simulink model "Quaternions_Method"  (R2021b)
settings: Solver=ode113  StartTime=0.0  StopTime=Time  RelTol=1e-13  AbsTol=1e-8
values from neighbouring files (symbols this model uses):
  a = 8.6251e+06    (= 8625100)    [Quaternions_method_parameters.m]    (also in car2kep.m = -(mu/(2*E)))
  A_MB = 0.5    [Quaternions_method_parameters.m]
  A_SP = 1    [Quaternions_method_parameters.m]
  c = 299792*10^3    (= 299792000)    [Quaternions_method_parameters.m]
  e = norm(e)    [Lab_7_task_1_4_parameters.m]    (also in Lab_7_task_5_parameters.m; Quaternions_method_parameters.m = 0.1195; car2kep.m = 1/mu * [((v_norm)^2 - (mu/r_norm)).*r - (dot(r, v).*v)])
  ii = 0.3815    [Quaternions_method_parameters.m]
  Ix = 0.04    [Quaternions_method_parameters.m]
  Iy = 0.06    [Quaternions_method_parameters.m]
  Iz = 0.08    [Quaternions_method_parameters.m]
  muP = astroConstants(13)*10^9    [Lab_7_task_1_4_parameters.m]    (also in Lab_7_task_5_parameters.m; Quaternions_method_parameters.m = 398527110340000)
  om_x = 1e-6    (= 1e-06)    [Quaternions_method_parameters.m]
  om_y = 1e-6    (= 1e-06)    [Quaternions_method_parameters.m]
  om_z = n    [Quaternions_method_parameters.m]
  omega_0 = [om_x, om_y, om_z]    [Quaternions_method_parameters.m]
  RS_MB = 0.5    [Quaternions_method_parameters.m]
  theta00 = 0    [Quaternions_method_parameters.m]
undefined symbols (not defined in the file or in its folder): I, Iinv, Rs_SP
libraries: vrlib x3, simulink_extras x1, robotcorelib x1
(part 2 of 2)

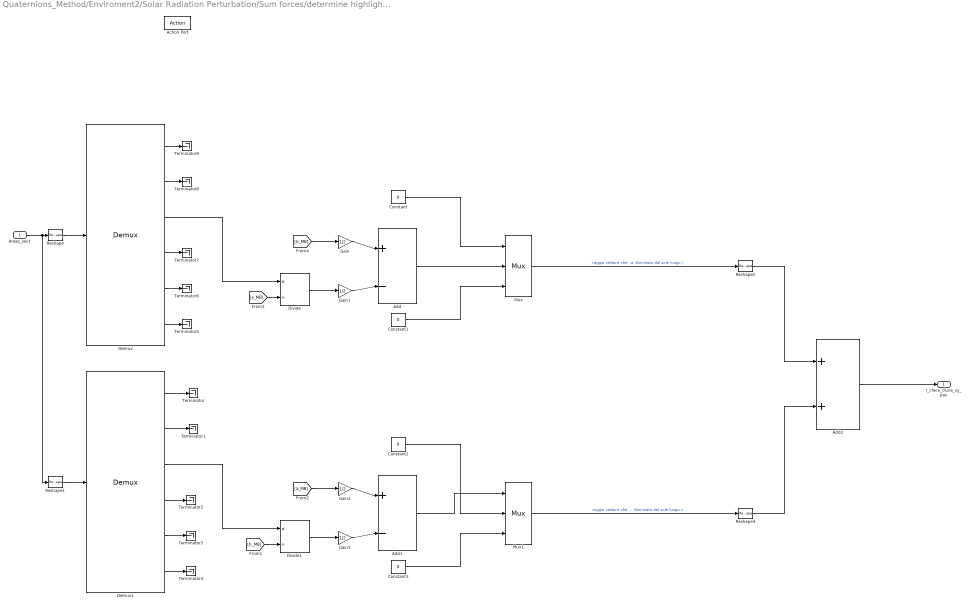
== system Quaternions_Method/Enviroment2/Solar Radiation Perturbation/Sum forces/determine highlighted area/creazione della matrice che ha per colonne i vettori distanza tra il CM del MB e i centri geom delle aree illuminate dal sole /If Action Subsystem ==
  Areas_vect : Inport
  Action Port : ActionPort  ActionPortLabel=if(u1>0 & u2>0)
  Add : Sum  Inputs=+|-
  Add1 : Sum  Inputs=+|-
  Add2 : Sum
  Constant{,1..3} (4 alike) : Constant  Value=0
  Demux : Demux  Outputs=6
  Demux1 : Demux  Outputs=6
  Divide : Product  Inputs=*/
  Divide1 : Product  Inputs=*/
  Gain{,1..3} (4 alike) : Gain  Gain=1/2
  Mux : Mux  Inputs=3
  Mux1 : Mux  Inputs=3
  Reshape{,1..3} (4 alike) : Reshape  OutputDimensionality=Column vector (2-D)
  Terminator{,1..9} (10 alike) : Terminator
  r_cface_cluce_xy_pos : Outport
  wires:
  Constant/1 -> Mux/1
  Add/1 -> Mux/2
  Divide/1 -> Gain1/1
  Mux/1 -> Reshape2/1  "raggio vettore che collega il centro geom della faccia con il centro geom della faccia illuminata dal sole lungo j"
  Gain1/1 -> Add/2
  Demux/3 -> Divide/1
  [b_MB] -> Gain/1
  Gain/1 -> Add/1
  [a_MB] -> Divide/2
  Areas_vect/1 -> Reshape1/1, Reshape/1
  Constant1/1 -> Mux/3
  Reshape/1 -> Demux/1
  Add1/1 -> Mux1/1
  [b_MB] -> Divide1/2
  Mux1/1 -> Reshape3/1  "raggio vettore che collega il centro geom della faccia con il centro geom della faccia illuminata dal sole lungo x"
  Constant2/1 -> Mux1/2
  Demux1/3 -> Divide1/1
  Constant3/1 -> Mux1/3
  Gain3/1 -> Add1/2
  Gain2/1 -> Add1/1
  Reshape1/1 -> Demux1/1
  Divide1/1 -> Gain3/1
  [a_MB] -> Gain2/1
  Reshape2/1 -> Add2/1
  Reshape3/1 -> Add2/2
  Add2/1 -> r_cface_cluce_xy_pos/1
  Demux1/1 -> Terminator/1
  Demux1/2 -> Terminator1/1
  Demux1/5 -> Terminator3/1
  Demux1/6 -> Terminator4/1
  Demux1/4 -> Terminator2/1
  Demux/6 -> Terminator5/1
  Demux/5 -> Terminator6/1
  Demux/4 -> Terminator7/1
  Demux/1 -> Terminator9/1
  Demux/2 -> Terminator8/1

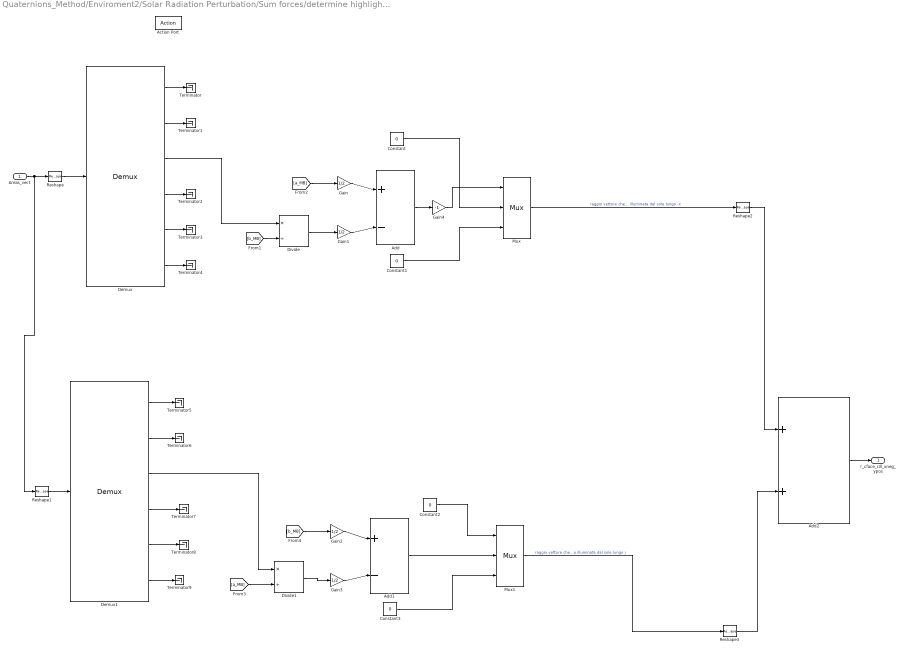
== system Quaternions_Method/Enviroment2/Solar Radiation Perturbation/Sum forces/determine highlighted area/creazione della matrice che ha per colonne i vettori distanza tra il CM del MB e i centri geom delle aree illuminate dal sole /If Action Subsystem1 ==
  Areas_vect : Inport
  Action Port : ActionPort  ActionPortLabel=if(u1<0 & u2>0)
  Add : Sum  Inputs=+|-
  Add1 : Sum  Inputs=+|-
  Add2 : Sum
  Constant{,1..3} (4 alike) : Constant  Value=0
  Demux : Demux  Outputs=6
  Demux1 : Demux  Outputs=6
  Divide : Product  Inputs=*/
  Divide1 : Product  Inputs=*/
  Gain{,1..3} (4 alike) : Gain  Gain=1/2
  Gain4 : Gain  Gain=-1
  Mux : Mux  Inputs=3
  Mux1 : Mux  Inputs=3
  Reshape{,1..3} (4 alike) : Reshape  OutputDimensionality=Column vector (2-D)
  Terminator{,1..9} (10 alike) : Terminator
  r_cface_cill_xneg_ypos : Outport
  wires:
  Reshape2/1 -> Add2/1
  Areas_vect/1 -> Reshape1/1, Reshape/1
  [b_MB] -> Divide/2
  Reshape/1 -> Demux/1
  [a_MB] -> Gain/1
  Gain/1 -> Add/1
  Gain1/1 -> Add/2
  Constant1/1 -> Mux/3
  Mux/1 -> Reshape2/1  "raggio vettore che collega il centro geom della faccia con il centro geom della faccia illuminata dal sole lungo -x"
  Demux/3 -> Divide/1
  Divide/1 -> Gain1/1
  Constant/1 -> Mux/2
  Reshape3/1 -> Add2/2
  Constant2/1 -> Mux1/1
  Gain2/1 -> Add1/1
  Gain3/1 -> Add1/2
  Mux1/1 -> Reshape3/1  "raggio vettore che collega il centro geom della faccia con il centro geom della faccia illuminata dal sole lungo j"
  Add1/1 -> Mux1/2
  Demux1/3 -> Divide1/1
  [a_MB] -> Divide1/2
  [b_MB] -> Gain2/1
  Divide1/1 -> Gain3/1
  Constant3/1 -> Mux1/3
  Add2/1 -> r_cface_cill_xneg_ypos/1
  Reshape1/1 -> Demux1/1
  Add/1 -> Gain4/1
  Gain4/1 -> Mux/1
  Demux/1 -> Terminator/1
  Demux/2 -> Terminator1/1
  Demux/4 -> Terminator2/1
  Demux/5 -> Terminator3/1
  Demux/6 -> Terminator4/1
  Demux1/1 -> Terminator5/1
  Demux1/2 -> Terminator6/1
  Demux1/4 -> Terminator7/1
  Demux1/5 -> Terminator8/1
  Demux1/6 -> Terminator9/1

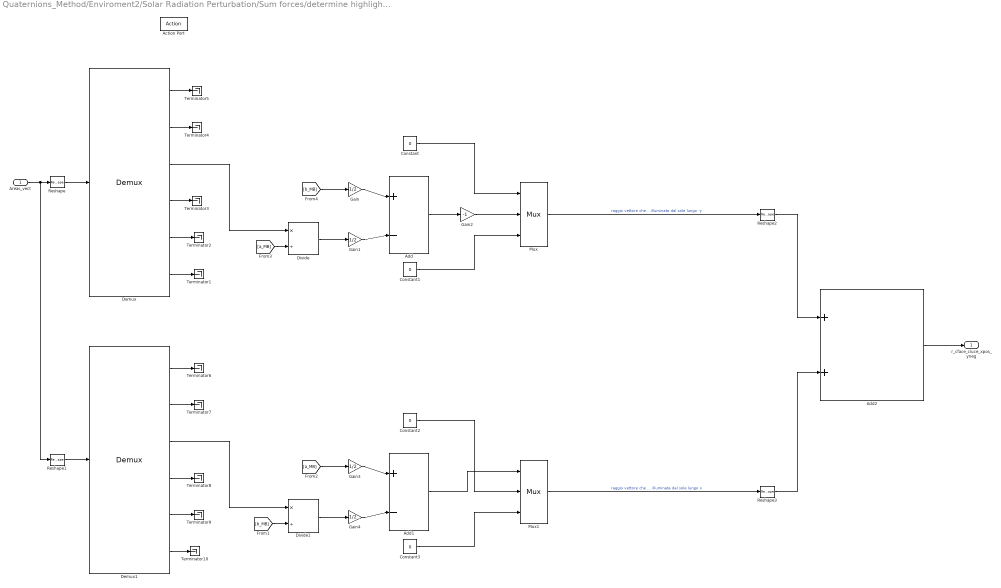
== system Quaternions_Method/Enviroment2/Solar Radiation Perturbation/Sum forces/determine highlighted area/creazione della matrice che ha per colonne i vettori distanza tra il CM del MB e i centri geom delle aree illuminate dal sole /If Action Subsystem2 ==
  Areas_vect : Inport
  Action Port : ActionPort  ActionPortLabel=if(u1>0 & u2<0)
  Add : Sum  Inputs=+|-
  Add1 : Sum  Inputs=+|-
  Add2 : Sum
  Constant{,1..3} (4 alike) : Constant  Value=0
  Demux : Demux  Outputs=6
  Demux1 : Demux  Outputs=6
  Divide : Product  Inputs=*/
  Divide1 : Product  Inputs=*/
  Gain{,1,3..4} (4 alike) : Gain  Gain=1/2
  Gain2 : Gain  Gain=-1
  Mux : Mux  Inputs=3
  Mux1 : Mux  Inputs=3
  Reshape{,1..3} (4 alike) : Reshape  OutputDimensionality=Column vector (2-D)
  Terminator{1..10} (10 alike) : Terminator
  r_cface_cluce_xpos_yneg : Outport
  wires:
  Divide/1 -> Gain1/1
  Demux/3 -> Divide/1
  Mux/1 -> Reshape2/1  "raggio vettore che collega il centro geom della faccia con il centro geom della faccia illuminata dal sole lungo -y"
  Constant1/1 -> Mux/3
  Gain1/1 -> Add/2
  Gain/1 -> Add/1
  [b_MB] -> Gain/1
  Reshape/1 -> Demux/1
  [a_MB] -> Divide/2
  Constant/1 -> Mux/1
  Add/1 -> Gain2/1
  Gain2/1 -> Mux/2
  Add1/1 -> Mux1/1
  Reshape1/1 -> Demux1/1
  [a_MB] -> Gain3/1
  Divide1/1 -> Gain4/1
  Gain3/1 -> Add1/1
  Gain4/1 -> Add1/2
  Demux1/3 -> Divide1/1
  Areas_vect/1 -> Reshape1/1, Reshape/1
  Mux1/1 -> Reshape3/1  "raggio vettore che collega il centro geom della faccia con il centro geom della faccia illuminata dal sole lungo x"
  [b_MB] -> Divide1/2
  Constant2/1 -> Mux1/2
  Constant3/1 -> Mux1/3
  Reshape2/1 -> Add2/1
  Reshape3/1 -> Add2/2
  Add2/1 -> r_cface_cluce_xpos_yneg/1
  Demux/6 -> Terminator1/1
  Demux/5 -> Terminator2/1
  Demux/4 -> Terminator3/1
  Demux/1 -> Terminator5/1
  Demux/2 -> Terminator4/1
  Demux1/1 -> Terminator6/1
  Demux1/2 -> Terminator7/1
  Demux1/4 -> Terminator8/1
  Demux1/5 -> Terminator9/1
  Demux1/6 -> Terminator10/1

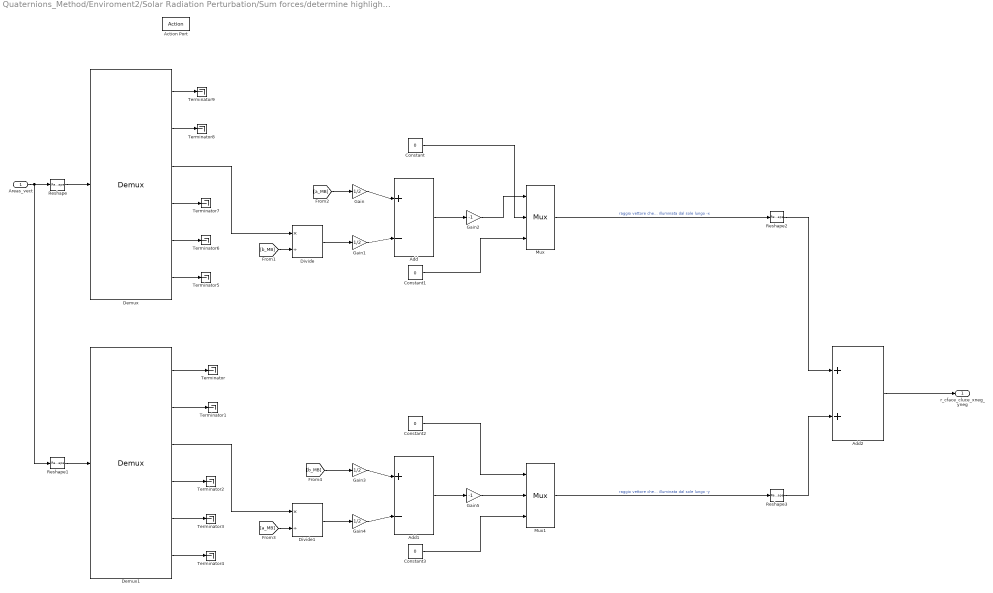
== system Quaternions_Method/Enviroment2/Solar Radiation Perturbation/Sum forces/determine highlighted area/creazione della matrice che ha per colonne i vettori distanza tra il CM del MB e i centri geom delle aree illuminate dal sole /If Action Subsystem3 ==
  Areas_vect : Inport
  Action Port : ActionPort  ActionPortLabel=if(u1<0 & u2<0)
  Add : Sum  Inputs=+|-
  Add1 : Sum  Inputs=+|-
  Add2 : Sum
  Constant{,1..3} (4 alike) : Constant  Value=0
  Demux : Demux  Outputs=6
  Demux1 : Demux  Outputs=6
  Divide : Product  Inputs=*/
  Divide1 : Product  Inputs=*/
  Gain{,1,3..4} (4 alike) : Gain  Gain=1/2
  Gain2 : Gain  Gain=-1
  Gain5 : Gain  Gain=-1
  Mux : Mux  Inputs=3
  Mux1 : Mux  Inputs=3
  Reshape{,1..3} (4 alike) : Reshape  OutputDimensionality=Column vector (2-D)
  Terminator{,1..9} (10 alike) : Terminator
  r_cface_cluce_xneg_yneg : Outport
  wires:
  Add/1 -> Gain2/1
  Areas_vect/1 -> Reshape1/1, Reshape/1
  [b_MB] -> Divide/2
  Reshape/1 -> Demux/1
  Gain/1 -> Add/1
  Gain1/1 -> Add/2
  Constant1/1 -> Mux/3
  Mux/1 -> Reshape2/1  "raggio vettore che collega il centro geom della faccia con il centro geom della faccia illuminata dal sole lungo -x"
  Demux/3 -> Divide/1
  Divide/1 -> Gain1/1
  [a_MB] -> Gain/1
  Gain2/1 -> Mux/1
  Constant/1 -> Mux/2
  Mux1/1 -> Reshape3/1  "raggio vettore che collega il centro geom della faccia con il centro geom della faccia illuminata dal sole lungo -y"
  Gain4/1 -> Add1/2
  Gain3/1 -> Add1/1
  Constant3/1 -> Mux1/3
  Reshape1/1 -> Demux1/1
  [b_MB] -> Gain3/1
  [a_MB] -> Divide1/2
  Demux1/3 -> Divide1/1
  Gain5/1 -> Mux1/2
  Constant2/1 -> Mux1/1
  Add1/1 -> Gain5/1
  Divide1/1 -> Gain4/1
  Reshape3/1 -> Add2/2
  Reshape2/1 -> Add2/1
  Add2/1 -> r_cface_cluce_xneg_yneg/1
  Demux1/1 -> Terminator/1
  Demux1/2 -> Terminator1/1
  Demux1/5 -> Terminator3/1
  Demux1/6 -> Terminator4/1
  Demux1/4 -> Terminator2/1
  Demux/6 -> Terminator5/1
  Demux/5 -> Terminator6/1
  Demux/4 -> Terminator7/1
  Demux/2 -> Terminator8/1
  Demux/1 -> Terminator9/1

== system Quaternions_Method/Enviroment2/Solar Radiation Perturbation/Sum forces/determine highlighted area/creazione della matrice che ha per colonne i vettori distanza tra il CM del MB e i centri geom delle aree illuminate dal sole /creating distance between cm MB and centro geom lato ==
  Constant : Constant  Value=0
  Constant1 : Constant  Value=0
  Mux : Mux  Inputs=3
  Reshape : Reshape  OutputDimensionality=Column vector (2-D)
  Out1 : Outport
  wires:
  Constant/1 -> Mux/1
  Constant1/1 -> Mux/2
  [h_MB] -> Mux/3
  Mux/1 -> Reshape/1
  Reshape/1 -> Out1/1

== matlab function Quaternions_Method/Kinematics2/Creazione quaternione/Creation matrix [OM] ==
  data: om_x input; OM output; om_y input; om_z input
function OM  = fcn(om_x, om_y, om_z)

OM = [0 om_z -om_y om_x; 
      -om_z 0 om_x om_y; 
      om_y -om_x 0 om_z;
      -om_x -om_y -om_z 0];

end
